simulink model "distffun"  (Simulink 3.00)
settings: Solver=ode45  SolverMode=SingleTasking  StartTime=0.0  StopTime=15  MaxStep=0.01  RelTol=1e-3  AbsTol=1e-3
settings Model: TimeSaveName=t  SaveOutput=off

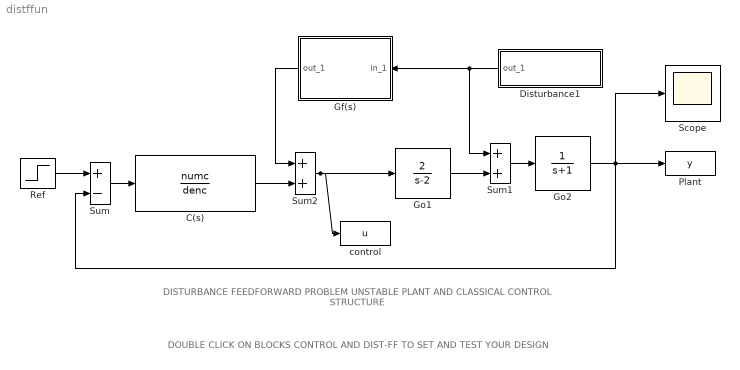
== system distffun ==
  note: DISTURBANCE FEEDFORWARD  PROBLEM
      | UNSTABLE PLANT AND CLASSICAL CONTROL STRUCTURE
  note: DOUBLE CLICK ON BLOCKS CONTROL AND DIST-FF TO SET AND TEST YOUR DESIGN
  C(s) : TransferFcn  Numerator=numc  Denominator=denc  mask(Controlador){@1=[38 88 72], @2=[1 13 0]}
      mask prompts: @1 "numerator:"; @2 "denominator:"
      mask help: Controlador
      mask init:
      | numc=@1;denc=@2;
      mask Help: Linear controller
      mask Display: disp('CONTROL')
  Disturbance1 : Subsystem  Orientation=left  mask(Generalised disturbance){@1=1, @2=0.5}
      mask prompts: @1 "Amplitude  of constant component:"; @2 "Amplitude  of varying component:"
      mask help: disturbance
      mask init:
      | Kc=@1;Kv=@2;
      mask Help: This block generates a signal with average value Kc and a varying component amplified by Kv
      mask Display: disp('Disturbance')
  Gf(s) : Subsystem  Orientation=left  mask(DIST-FF){@1=[-1 2], @2=[0.02  2]}
      mask prompts: @1 "numerator:"; @2 "denominator:"
      mask help: Disturbance feedforward block Gf
      mask init:
      | ngf=-@1;dgf=@2;
      mask Help: Dynamic controller to provide disturbance feedforward
      mask Display: disp('DIST-FF')
  Go1 : TransferFcn  Numerator=[2]  Denominator=[1 -2]
  Go2 : TransferFcn  Numerator=[1]  Denominator=[1 1]
  Plant : ToWorkspace  VariableName=y  SampleTime=0  SaveFormat=Matrix
      settings: Buffer=6000
  Ref : Step  Time=1  Before=0  After=1  SampleTime=0
  Scope : Scope
      settings: TickLabels=on  TimeRange=15.000000  YMin=-2  YMax=2  SaveToWorkspace=off  SaveName=ScopeData  DataFormat=Matrix
  Sum : Sum  Inputs=+-  SaturateOnIntegerOverflow=on
  Sum1 : Sum  Inputs=++  SaturateOnIntegerOverflow=on
  Sum2 : Sum  Inputs=++  SaturateOnIntegerOverflow=on
  control : ToWorkspace  VariableName=u  SampleTime=0  SaveFormat=Matrix
      settings: Buffer=6000
  wires:
  Sum/1 -> C(s)/1
  C(s)/1 -> Sum2/2
  Go1/1 -> Sum1/2
  Sum1/1 -> Go2/1
  Ref/1 -> Sum/1
  Gf(s)/1(out_1) -> Sum2/1
  Disturbance1/1(out_1) -> Sum1/1, Gf(s)/1(in_1)
  Sum2/1 -> Go1/1, control/1
  Go2/1 -> Plant/1, Sum/2, Scope/1

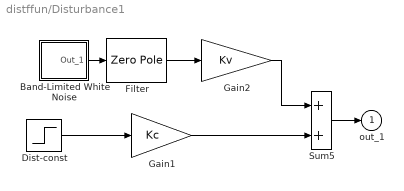
== system distffun/Disturbance1 ==
  Band-Limited White Noise : Subsystem  mask(Continuous White Noise.){@1=[0.1], @2=0.1, @3=[23341]}
      mask prompts: @1 "Noise Power:"; @2 "Sample Time:"; @3 "Seed"
      mask help:
      | White noise for continuous (s-domain) systems.
      | Band-limited using zero-order-hold.
      mask init:
      | Cov = @1; Ts = @2; seed = @3; r = rand(1,12); r2 = [r(1),r;r,r(12)]; t =[1:13;1:13];
      mask Help: Implemented using white noise into Zero-Order Hold block. The seed and power can be vectors of the same length to produce a vector of white noise sources. For faster simulation, set sample time to the highest value possible but in accordance with the fastest dynamics of system.
      mask Display: plot(t(:),r2(:))
  Dist-const : Step  Time=0  Before=0  After=1  SampleTime=0
  Filter : ZeroPole  Zeros=z  Poles=p  Gain=k  mask(buttap){@1=4, @2=6}
      mask prompts: @1 "Cutoff frequency (rad/sec)"; @2 "Order"
      mask help:
      | Analog Butterworth low pass filter.
      |
      | (Requires Signal Processing Toolbox)
      mask init:
      | [z,p,k]=buttap(@2); z=@1*z; p=@1*p; k=real(prod(-p)); [num,den]=zp2tf(z,p,k); w=logspace(log10(@1/10),log10(10*@1),20); h=freqs(num,den,w);
      mask Help: Butterworth low pass filter using MATLAB's butter command.
      mask Display: plot(20*log10(w),20*log10(abs(h)))
  Gain1 : Gain  Gain=Kc  SaturateOnIntegerOverflow=on
  Gain2 : Gain  Gain=Kv  SaturateOnIntegerOverflow=on
  Sum5 : Sum  Inputs=++  SaturateOnIntegerOverflow=on
  out_1 : Outport  Port=1  InitialOutput=0
  wires:
  Dist-const/1 -> Gain1/1
  Sum5/1 -> out_1/1
  Band-Limited White Noise/1(Out_1) -> Filter/1
  Gain1/1 -> Sum5/2
  Filter/1 -> Gain2/1
  Gain2/1 -> Sum5/1

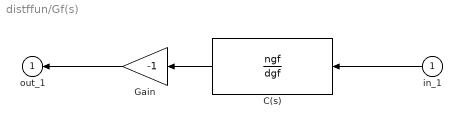
== system distffun/Gf(s) ==
  in_1 : Inport  Orientation=left  Port=1  PortWidth=-1  SampleTime=-1  DataType=auto
      settings: SignalType=auto
  C(s) : TransferFcn  Orientation=left  Numerator=ngf  Denominator=dgf
  Gain : Gain  Orientation=left  Gain=-1  SaturateOnIntegerOverflow=on
  out_1 : Outport  Orientation=left  Port=1  InitialOutput=0
  wires:
  Gain/1 -> out_1/1
  C(s)/1 -> Gain/1
  in_1/1 -> C(s)/1

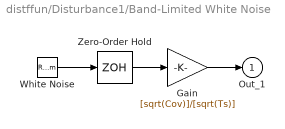
== system distffun/Disturbance1/Band-Limited White Noise ==
  Gain : Gain  Gain=[sqrt(Cov)]/[sqrt(Ts)]  SaturateOnIntegerOverflow=on
  White Noise : RandomNumber  Mean=0  Variance=1  Seed=seed  SampleTime=0
  Zero-Order Hold : ZeroOrderHold  SampleTime=Ts
  Out_1 : Outport  Port=1  InitialOutput=0
  wires:
  Zero-Order Hold/1 -> Gain/1
  Gain/1 -> Out_1/1
  White Noise/1 -> Zero-Order Hold/1
